simulink model "DPF_warning_lamp"  (R2019a)
settings: Solver=VariableStepAuto  StartTime=0.0  StopTime=100  RelTol=1e-3
undefined symbols (not defined in the file or in its folder): dpf_pressure
libraries: simulink x1
settings Model: DataDictionary=out7.sldd  Creator=admin  LastModifiedBy=admin

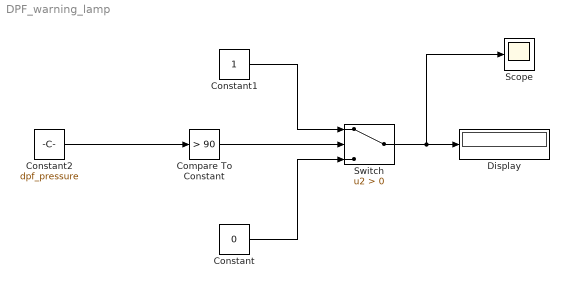
== system DPF_warning_lamp ==
  Compare To Constant : simulink/Logic and Bit Operations/Compare To Constant  relop=>  const=90  OutDataTypeStr=boolean
  Constant : Constant  Value=0
  Constant1 : Constant
  Constant2 : Constant  Value=dpf_pressure
  Display : Display
  Scope : Scope
  Switch : Switch  Criteria=u2 > Threshold
  wires:
  Compare To Constant/1 -> Switch/2
  Constant1/1 -> Switch/1
  Constant2/1 -> Compare To Constant/1
  Constant/1 -> Switch/3
  Switch/1 -> Scope/1, Display/1
